simulink model "simlation"  (R2019a)
settings: Solver=VariableStepAuto  StartTime=0.0  StopTime=10.0  RelTol=1e-3
undefined symbols (not defined in the file): DiscIntNeverNeededParam, kt, kx, ky
libraries: discretizing x8, simulink x4
settings Model: Creator=robot  LastModifiedBy=robot
settings OptimizationCC: DefaultParameterBehavior=Inlined  UseDivisionForNetSlopeComputation=on  GainParamInheritBuiltInType=on  UseFloatMulNetSlope=on  InlineInvariantSignals=on  PassReuseOutputArgsAs=Individual arguments  ZeroExternalMemoryAtStartup=off  ZeroInternalMemoryAtStartup=off  NoFixptDivByZeroProtection=on  EfficientFloat2IntCast=on  LifeSpan=1  OptimizeBlockOrder=speed  DifferentSizesBufferReuse=on
settings DebuggingCC: ParameterTunabilityLossMsg=error
settings HardwareCC: ProdBitPerInt=16  ProdBitPerPointer=16  ProdBitPerSizeT=16  ProdBitPerPtrDiffT=16  ProdLargestAtomicFloat=None  ProdWordSize=16  ProdLongLongMode=on  ProdHWDeviceType=STMicroelectronics->ST10/Super10
settings SFSimCC: MATLABDynamicMemAlloc=off
settings RTWCC: SystemTargetFile=ert.tlc  PackageGeneratedCodeAndArtifacts=on  PackageName=PathFollowing  TemplateMakefile=ert_default_tmf  GenerateReport=on  Toolchain=GNU Tools for ARM Embedded Processors  IncludeHyperlinkInReport=on  LaunchReport=on  GenerateTraceInfo=on  GenerateTraceReport=on  GenerateTraceReportSl=on  GenerateTraceReportSf=on  GenerateTraceReportEml=on  GenerateCodeMetricsReport=on
settings CodeAppCC: ForceParamTrailComments=on  IgnoreCustomStorageClasses=off  OperatorAnnotations=on  SimulinkDataObjDesc=on  SFDataObjDesc=on  CustomSymbolStrGlobalVar=rt$N$M  CustomSymbolStrType=$N$M  CustomSymbolStrFcn=$N$M$F  CustomSymbolStrMacro=$N$M  InsertBlockDesc=on
settings ERTTargetCC: TargetLangStandard=C99 (ISO)  GenerateSampleERTMain=on  IncludeMdlTerminateFcn=off  CombineSignalStateStructs=on  SupportComplex=off  SupportNonInlinedSFcns=on  InlinedParameterPlacement=NonHierarchical  ERTCustomFileTemplate=example_file_process.tlc  ERTFilePackagingFormat=CompactWithDataFile

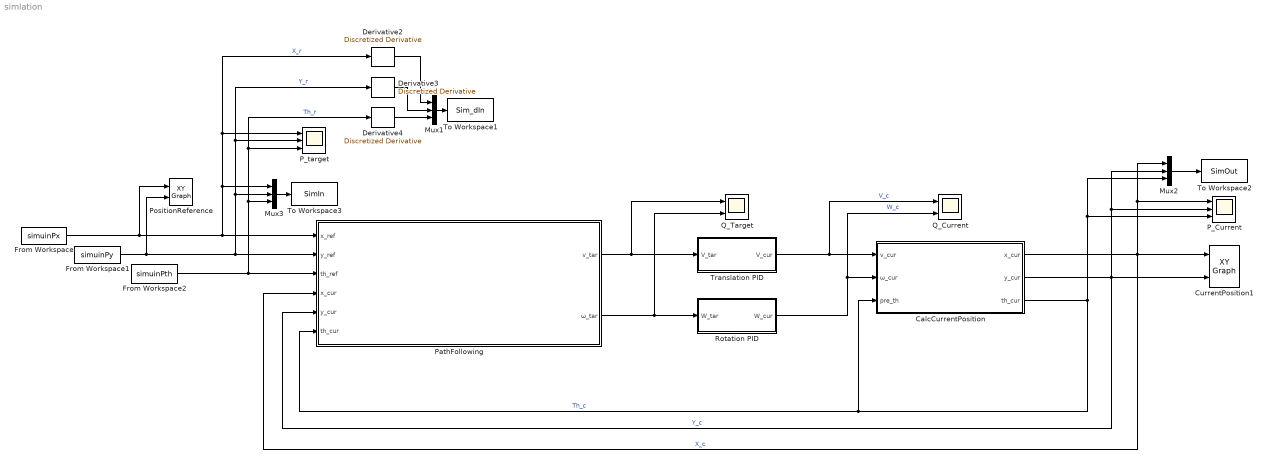
== system simlation ==
  "CalcCurrentPosition " : Subsystem
  CurrentPosition1 : simulink/Sinks/XY Graph  xmin=-200  xmax=200  ymin=-10  ymax=400  st=-1
  Derivative2 : discretizing/Discretized Derivative  method=tustin  SampleTime=0.01  Wc=1
      settings: SourceProductName=Simulink  SourceProductBaseCode=SL
  Derivative3 : discretizing/Discretized Derivative  method=tustin  SampleTime=0.01  Wc=1
      settings: SourceProductName=Simulink  SourceProductBaseCode=SL
  Derivative4 : discretizing/Discretized Derivative  method=tustin  SampleTime=0.01  Wc=1
      settings: SourceProductName=Simulink  SourceProductBaseCode=SL
  From Workspace : FromWorkspace  VariableName=simuinPx  SampleTime=0.01  mask(DiscretizedSource){}
      mask init:
      | %zoh
  From Workspace1 : FromWorkspace  VariableName=simuinPy  SampleTime=0.01  mask(DiscretizedSource){}
      mask init:
      | %zoh
  From Workspace2 : FromWorkspace  VariableName=simuinPth  SampleTime=0.01  mask(DiscretizedSource){}
      mask init:
      | %zoh
  Mux1 : Mux  Inputs=3
  Mux2 : Mux  Inputs=3
  Mux3 : Mux  Inputs=3
  P_Current : Scope  NumInputPorts=3
  P_target : Scope  NumInputPorts=3
  PathFollowing : Subsystem  TreatAsAtomicUnit=on
  PositionReference : simulink/Sinks/XY Graph  xmin=-200  xmax=200  ymin=-10  ymax=400  st=-1
  Q_Current : Scope  NumInputPorts=2
  Q_Target : Scope  NumInputPorts=2
  Rotation PID : Subsystem
  To Workspace1 : ToWorkspace  VariableName=Sim_dIn  SampleTime=-1
  To Workspace2 : ToWorkspace  VariableName=SimOut  SampleTime=-1
  To Workspace3 : ToWorkspace  VariableName=SimIn  SampleTime=-1
  Translation PID : Subsystem  TreatAsAtomicUnit=on
  wires:
  "CalcCurrentPosition "/3(th_cur) -> "CalcCurrentPosition "/3(pre_th), PathFollowing/6(th_cur), Mux2/3, P_Current/3  "Th_c"
  "CalcCurrentPosition "/1(x_cur) -> PathFollowing/4("x_cur "), CurrentPosition1/1, Mux2/1, P_Current/1  "X_c"
  Mux3/1 -> To Workspace3/1
  From Workspace/1 -> PathFollowing/1(x_ref), P_target/1, Derivative2/1, Mux3/1, PositionReference/1  "X_r"
  Mux2/1 -> To Workspace2/1
  From Workspace2/1 -> PathFollowing/3("th_ref "), Derivative4/1, P_target/3, Mux3/3  "Th_r"
  Mux1/1 -> To Workspace1/1
  "CalcCurrentPosition "/2(y_cur) -> Mux2/2, P_Current/2, CurrentPosition1/2, PathFollowing/5(y_cur)  "Y_c"
  Derivative2/1 -> Mux1/1
  From Workspace1/1 -> PathFollowing/2(y_ref), Derivative3/1, P_target/2, Mux3/2, PositionReference/2  "Y_r"
  Derivative3/1 -> Mux1/2
  Translation PID/1(V_cur) -> "CalcCurrentPosition "/1(v_cur), Q_Current/1  "V_c"
  Derivative4/1 -> Mux1/3
  PathFollowing/2(ω_tar) -> Rotation PID/1(W_tar), Q_Target/2
  PathFollowing/1(v_tar) -> Translation PID/1(V_tar), Q_Target/1
  Rotation PID/1(W_cur) -> "CalcCurrentPosition "/2(ω_cur), Q_Current/2  "W_c"

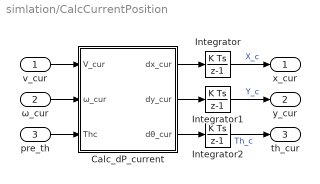
== system simlation/CalcCurrentPosition  ==
  v_cur : Inport
  ω_cur : Inport  Port=2
  pre_th : Inport  Port=3
  Calc_dP_current : Subsystem
  Integrator : DiscreteIntegrator  SampleTime=0.01  ICPrevOutput=DiscIntNeverNeededParam  ICPrevScaledInput=DiscIntNeverNeededParam  mask(DiscretizedDiscreteIntegrator){}
      mask init:
      | %zoh
  Integrator1 : DiscreteIntegrator  SampleTime=0.01  ICPrevOutput=DiscIntNeverNeededParam  ICPrevScaledInput=DiscIntNeverNeededParam  mask(DiscretizedDiscreteIntegrator){}
      mask init:
      | %zoh
  Integrator2 : DiscreteIntegrator  SampleTime=0.01  ICPrevOutput=DiscIntNeverNeededParam  ICPrevScaledInput=DiscIntNeverNeededParam  mask(DiscretizedDiscreteIntegrator){}
      mask init:
      | %zoh
  x_cur : Outport
  y_cur : Outport  Port=2
  th_cur : Outport  Port=3
  wires:
  ω_cur/1 -> Calc_dP_current/2(ω_cur)
  v_cur/1 -> Calc_dP_current/1(V_cur)
  pre_th/1 -> Calc_dP_current/3(Thc)
  Integrator/1 -> x_cur/1  "X_c"
  Calc_dP_current/1(dx_cur) -> Integrator/1
  Calc_dP_current/2(dy_cur) -> Integrator1/1
  Calc_dP_current/3(dθ_cur) -> Integrator2/1
  Integrator2/1 -> th_cur/1  "Th_c"
  Integrator1/1 -> y_cur/1  "Y_c"

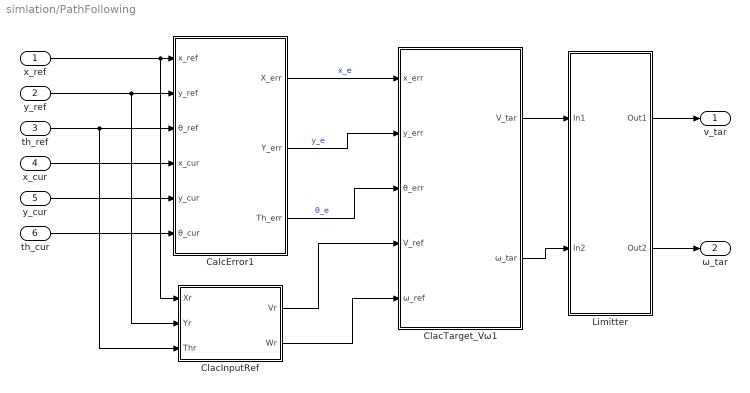
== system simlation/PathFollowing ==
  x_ref : Inport
  y_ref : Inport  Port=2
  "th_ref " : Inport  Port=3
  "x_cur " : Inport  Port=4
  y_cur : Inport  Port=5
  th_cur : Inport  Port=6
  CalcError1 : Subsystem  TreatAsAtomicUnit=on
      settings: RTWSystemCode=Nonreusable function
  "ClacInputRef " : Subsystem  TreatAsAtomicUnit=on
  ClacTarget_Vω1 : Subsystem  TreatAsAtomicUnit=on
  Limitter : Subsystem  TreatAsAtomicUnit=on
  v_tar : Outport
  ω_tar : Outport  Port=2
  wires:
  x_ref/1 -> "ClacInputRef "/1(Xr), CalcError1/1(x_ref)
  y_ref/1 -> CalcError1/2(y_ref), "ClacInputRef "/2(Yr)
  "th_ref "/1 -> "ClacInputRef "/3(Thr), CalcError1/3(θ_ref)
  CalcError1/1(X_err) -> ClacTarget_Vω1/1(x_err)  "x_e"
  CalcError1/2(Y_err) -> ClacTarget_Vω1/2(y_err)  "y_e"
  CalcError1/3(Th_err) -> ClacTarget_Vω1/3(θ_err)  "θ_e"
  "ClacInputRef "/1(Vr) -> ClacTarget_Vω1/4(V_ref)
  "ClacInputRef "/2(Wr) -> ClacTarget_Vω1/5(ω_ref)
  ClacTarget_Vω1/1(V_tar) -> Limitter/1(In1)
  ClacTarget_Vω1/2(ω_tar) -> Limitter/2(In2)
  Limitter/1(Out1) -> v_tar/1
  Limitter/2(Out2) -> ω_tar/1
  "x_cur "/1 -> CalcError1/4(x_cur)
  y_cur/1 -> CalcError1/5(y_cur)
  th_cur/1 -> CalcError1/6(θ_cur)

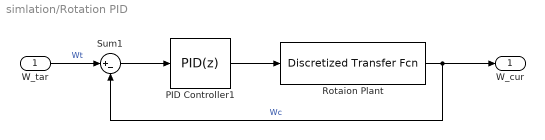
== system simlation/Rotation PID ==
  W_tar : Inport
  PID Controller1 : simulink/Continuous/PID Controller  Controller=PID  Form=Parallel  TimeDomain=Discrete-time  SampleTime=0.001  IntegratorMethod=Forward Euler  FilterMethod=Forward Euler  ControllerParametersSource=internal  P=-218.8515  I=-4309.9877  D=0  UseFilter=on  N=100  TunerSelectOption=Transfer Function Based (PID Tuner App)  InitialConditionSource=internal  InitialConditionForIntegrator=0  InitialConditionForFilter=0  DifferentiatorICPrevScaledInput=0  ExternalReset=none  TrackingMode=off  Kt=1  LimitOutput=on  UpperSaturationLimit=1200  LowerSaturationLimit=-1200  LinearizeAsGain=on  AntiWindupMode=none  Kb=1  POutMin=[]  POutMax=[]  IOutMin=[]  IOutMax=[]  DOutMin=[]  DOutMax=[]  NOutMin=[]  NOutMax=[]  SumOutMin=[]  SumOutMax=[]  SaturationOutMin=[]  SaturationOutMax=[]  PParamMin=[]  PParamMax=[]  IParamMin=[]  IParamMax=[]  DParamMin=[]  DParamMax=[]  NParamMin=[]  NParamMax=[]  KbParamMin=[]  KbParamMax=[]  KtParamMin=[]  KtParamMax=[]  KbOutMin=[]  KbOutMax=[]  KtOutMin=[]  KtOutMax=[]  IntegratorOutMin=[]  IntegratorOutMax=[]  FilterOutMin=[]  FilterOutMax=[]  SumI1OutMin=[]  SumI1OutMax=[]  SumI2OutMin=[]  SumI2OutMax=[]  SumI3OutMin=[]  SumI3OutMax=[]  SumI4OutMin=[]  SumI4OutMax=[]  SumDOutMin=[]  SumDOutMax=[]  DifferentiatorOutMin=[]  DifferentiatorOutMax=[]  FilterDiffOutCoefMin=[]  FilterDiffOutCoefMax=[]  ReciprocalOutMin=[]  ReciprocalOutMax=[]  SumDenOutMin=[]  SumDenOutMax=[]  SumNumOutMin=[]  SumNumOutMax=[]  DivideOutMin=[]  DivideOutMax=[]  IntegratorContinuousStateAttributes=''  IntegratorStateMustResolveToSignalObject=off  IntegratorRTWStateStorageClass=Auto  FilterContinuousStateAttributes=''  FilterStateMustResolveToSignalObject=off  FilterRTWStateStorageClass=Auto  ParallelPVariant=InternalParameters  IdealPVariant=Disabled  IVariant=InternalParameters  DVariant=InternalParameters  IntegratorVariant=Discrete  SatVariant=Enabled  AWVariant=Passthrough  PCopyVariant=Disabled  TRVariant=Disabled  FdbkBlocksVariant=Forward  IdealPFdbkVariant=Disabled  SatFdbkVariant=Disabled  DerivativeFilterVariant=ForwardEulerFilter  NVariant=InternalParameters  NCopyVariant=Disabled  FilterICVariant=InternalICsFilter  IntegratorICVariant=InternalICs  ExternalResetVariant=Disabled  TRSumVariant=Passthrough  SumFdbkVariant=Disabled  SumVariant=Sum_PID
  Rotaion Plant : discretizing/Discretized Transfer Fcn  Numerator=[-0.4447 -7.13]  Denominator=[1 36.42 145.2]  AbsTol=auto  SampleTime=0.01  method=zoh  Wc=1
      settings: SourceProductName=Simulink  SourceProductBaseCode=SL
  Sum1 : Sum  Inputs=|+-
  W_cur : Outport
  wires:
  PID Controller1/1 -> Rotaion Plant/1
  Sum1/1 -> PID Controller1/1
  W_tar/1 -> Sum1/1  "Wt"
  Rotaion Plant/1 -> Sum1/2, W_cur/1  "Wc"

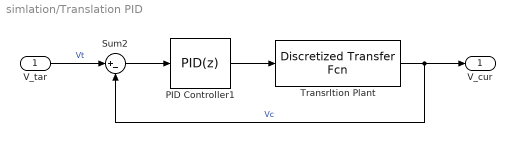
== system simlation/Translation PID ==
  V_tar : Inport
  PID Controller1 : simulink/Continuous/PID Controller  Controller=PID  Form=Parallel  TimeDomain=Discrete-time  SampleTime=0.001  IntegratorMethod=Forward Euler  FilterMethod=Forward Euler  ControllerParametersSource=internal  P=0.73598  I=3.7518  D=0  UseFilter=on  N=100  TunerSelectOption=Transfer Function Based (PID Tuner App)  InitialConditionSource=internal  InitialConditionForIntegrator=0  InitialConditionForFilter=0  DifferentiatorICPrevScaledInput=0  ExternalReset=none  TrackingMode=off  Kt=1  LimitOutput=on  UpperSaturationLimit=1200  LowerSaturationLimit=-1200  LinearizeAsGain=on  AntiWindupMode=none  Kb=1  POutMin=[]  POutMax=[]  IOutMin=[]  IOutMax=[]  DOutMin=[]  DOutMax=[]  NOutMin=[]  NOutMax=[]  SumOutMin=[]  SumOutMax=[]  SaturationOutMin=[]  SaturationOutMax=[]  PParamMin=[]  PParamMax=[]  IParamMin=[]  IParamMax=[]  DParamMin=[]  DParamMax=[]  NParamMin=[]  NParamMax=[]  KbParamMin=[]  KbParamMax=[]  KtParamMin=[]  KtParamMax=[]  KbOutMin=[]  KbOutMax=[]  KtOutMin=[]  KtOutMax=[]  IntegratorOutMin=[]  IntegratorOutMax=[]  FilterOutMin=[]  FilterOutMax=[]  SumI1OutMin=[]  SumI1OutMax=[]  SumI2OutMin=[]  SumI2OutMax=[]  SumI3OutMin=[]  SumI3OutMax=[]  SumI4OutMin=[]  SumI4OutMax=[]  SumDOutMin=[]  SumDOutMax=[]  DifferentiatorOutMin=[]  DifferentiatorOutMax=[]  FilterDiffOutCoefMin=[]  FilterDiffOutCoefMax=[]  ReciprocalOutMin=[]  ReciprocalOutMax=[]  SumDenOutMin=[]  SumDenOutMax=[]  SumNumOutMin=[]  SumNumOutMax=[]  DivideOutMin=[]  DivideOutMax=[]  IntegratorContinuousStateAttributes=''  IntegratorStateMustResolveToSignalObject=off  IntegratorRTWStateStorageClass=Auto  FilterContinuousStateAttributes=''  FilterStateMustResolveToSignalObject=off  FilterRTWStateStorageClass=Auto  ParallelPVariant=InternalParameters  IdealPVariant=Disabled  IVariant=InternalParameters  DVariant=InternalParameters  IntegratorVariant=Discrete  SatVariant=Enabled  AWVariant=Passthrough  PCopyVariant=Disabled  TRVariant=Disabled  FdbkBlocksVariant=Forward  IdealPFdbkVariant=Disabled  SatFdbkVariant=Disabled  DerivativeFilterVariant=ForwardEulerFilter  NVariant=InternalParameters  NCopyVariant=Disabled  FilterICVariant=InternalICsFilter  IntegratorICVariant=InternalICs  ExternalResetVariant=Disabled  TRSumVariant=Passthrough  SumFdbkVariant=Disabled  SumVariant=Sum_PID
  Sum2 : Sum  Inputs=|+-
  Transrltion Plant : discretizing/Discretized Transfer Fcn  Numerator=[353.7 1.175e04]  Denominator=[1 1042 1788]  AbsTol=auto  SampleTime=0.01  method=zoh  Wc=1
      settings: SourceProductName=Simulink  SourceProductBaseCode=SL
  V_cur : Outport
  wires:
  Sum2/1 -> PID Controller1/1
  PID Controller1/1 -> Transrltion Plant/1
  Transrltion Plant/1 -> V_cur/1, Sum2/2  "Vc"
  V_tar/1 -> Sum2/1  "Vt"

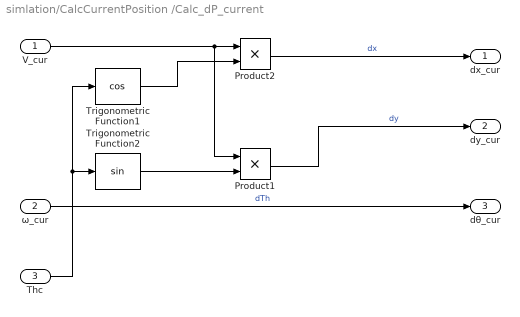
== system simlation/CalcCurrentPosition /Calc_dP_current ==
  V_cur : Inport
  ω_cur : Inport  Port=2
  Thc : Inport  Port=3
  Product1 : Product
  Product2 : Product
  Trigonometric Function1 : Trigonometry  Operator=cos
  Trigonometric Function2 : Trigonometry
  dx_cur : Outport
  dy_cur : Outport  Port=2
  dθ_cur : Outport  Port=3
  wires:
  V_cur/1 -> Product2/1, Product1/1
  Trigonometric Function1/1 -> Product2/2
  Thc/1 -> Trigonometric Function2/1, Trigonometric Function1/1
  Product2/1 -> dx_cur/1  "dx"
  Product1/1 -> dy_cur/1  "dy"
  Trigonometric Function2/1 -> Product1/2
  ω_cur/1 -> dθ_cur/1  "dTh"

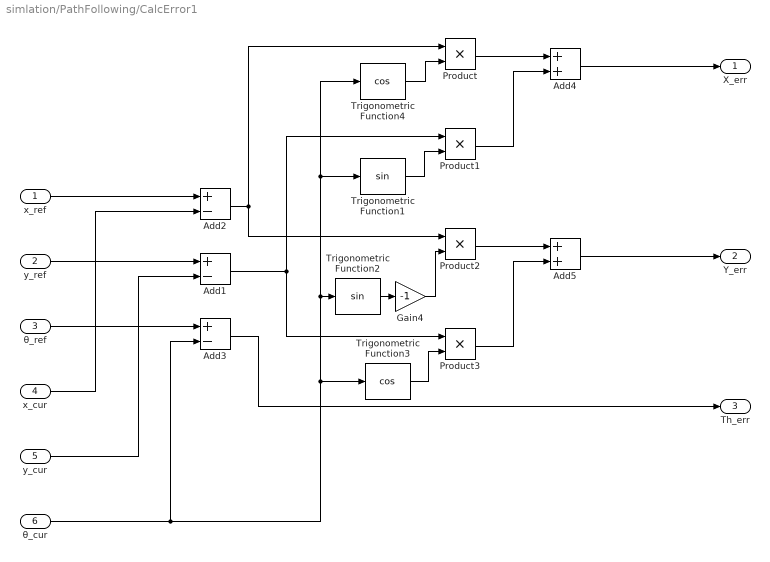
== system simlation/PathFollowing/CalcError1 ==
  x_ref : Inport
  y_ref : Inport  Port=2
  θ_ref : Inport  Port=3
  x_cur : Inport  Port=4
  y_cur : Inport  Port=5
  θ_cur : Inport  Port=6
  Add1 : Sum  Inputs=+-
  Add2 : Sum  Inputs=+-
  Add3 : Sum  Inputs=+-
  Add4 : Sum
  Add5 : Sum
  Gain4 : Gain  Gain=-1
  Product{,1..3} (4 alike) : Product
  Trigonometric Function1 : Trigonometry
  Trigonometric Function2 : Trigonometry
  Trigonometric Function3 : Trigonometry  Operator=cos
  Trigonometric Function4 : Trigonometry  Operator=cos
  X_err : Outport
  Y_err : Outport  Port=2
  Th_err : Outport  Port=3
  wires:
  x_cur/1 -> Add2/2
  x_ref/1 -> Add2/1
  y_ref/1 -> Add1/1
  y_cur/1 -> Add1/2
  θ_cur/1 -> Trigonometric Function4/1, Trigonometric Function1/1, Trigonometric Function2/1, Trigonometric Function3/1, Add3/2
  Trigonometric Function4/1 -> Product/2
  Product/1 -> Add4/1
  Trigonometric Function1/1 -> Product1/2
  Add1/1 -> Product3/1, Product1/1
  Product1/1 -> Add4/2
  Add4/1 -> X_err/1
  Add3/1 -> Th_err/1
  Add2/1 -> Product2/1, Product/1
  Product2/1 -> Add5/1
  Trigonometric Function3/1 -> Product3/2
  Product3/1 -> Add5/2
  Add5/1 -> Y_err/1
  Trigonometric Function2/1 -> Gain4/1
  Gain4/1 -> Product2/2
  θ_ref/1 -> Add3/1

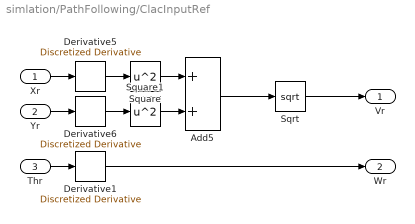
== system simlation/PathFollowing/ClacInputRef  ==
  Xr : Inport
  Yr : Inport  Port=2
  Thr : Inport  Port=3
  Add5 : Sum
  Derivative1 : discretizing/Discretized Derivative  method=tustin  SampleTime=0.01  Wc=1
      settings: SourceProductName=Simulink  SourceProductBaseCode=SL
  Derivative5 : discretizing/Discretized Derivative  method=tustin  SampleTime=0.01  Wc=1
      settings: SourceProductName=Simulink  SourceProductBaseCode=SL
  Derivative6 : discretizing/Discretized Derivative  method=tustin  SampleTime=0.01  Wc=1
      settings: SourceProductName=Simulink  SourceProductBaseCode=SL
  Sqrt : Sqrt  SaturateOnIntegerOverflow=on
  Square : Math  Operator=square  SaturateOnIntegerOverflow=on
  Square1 : Math  Operator=square  SaturateOnIntegerOverflow=on
  Vr : Outport
  Wr : Outport  Port=2
  wires:
  Sqrt/1 -> Vr/1
  Square1/1 -> Add5/2
  Derivative1/1 -> Wr/1
  Square/1 -> Add5/1
  Add5/1 -> Sqrt/1
  Derivative6/1 -> Square1/1
  Derivative5/1 -> Square/1
  Xr/1 -> Derivative5/1
  Yr/1 -> Derivative6/1
  Thr/1 -> Derivative1/1

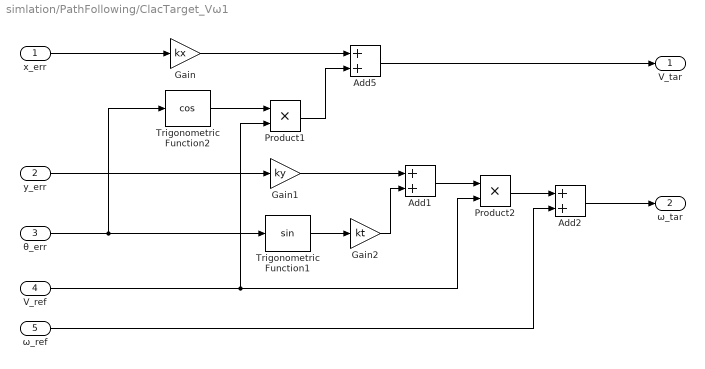
== system simlation/PathFollowing/ClacTarget_Vω1 ==
  x_err : Inport
  y_err : Inport  Port=2
  θ_err : Inport  Port=3
  V_ref : Inport  Port=4
  ω_ref : Inport  Port=5
  Add1 : Sum
  Add2 : Sum
  Add5 : Sum
  Gain : Gain  Gain=kx
  Gain1 : Gain  Gain=ky
  Gain2 : Gain  Gain=kt
  Product1 : Product
  Product2 : Product
  Trigonometric Function1 : Trigonometry
  Trigonometric Function2 : Trigonometry  Operator=cos
  V_tar : Outport
  ω_tar : Outport  Port=2
  wires:
  x_err/1 -> Gain/1
  Gain/1 -> Add5/1
  θ_err/1 -> Trigonometric Function1/1, Trigonometric Function2/1
  Trigonometric Function2/1 -> Product1/1
  V_ref/1 -> Product2/2, Product1/2
  Product1/1 -> Add5/2
  Add5/1 -> V_tar/1
  y_err/1 -> Gain1/1
  Gain1/1 -> Add1/1
  Trigonometric Function1/1 -> Gain2/1
  Gain2/1 -> Add1/2
  Add1/1 -> Product2/1
  Product2/1 -> Add2/1
  ω_ref/1 -> Add2/2
  Add2/1 -> ω_tar/1

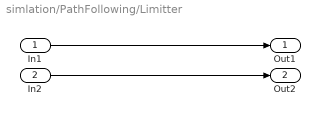
== system simlation/PathFollowing/Limitter ==
  In1 : Inport
  In2 : Inport  Port=2
  Out1 : Outport
  Out2 : Outport  Port=2
  wires:
  In1/1 -> Out1/1
  In2/1 -> Out2/1
